simulink model "ex2_model"  (R2013a)
settings: Solver=ode45  StartTime=0.0  StopTime=10.0  RelTol=1e-3
values from neighbouring files (symbols this model uses):
  q_0 = 0    [ex6.m]
  q_dot_0 = 0    [ex6.m]
undefined symbols (not defined in the file or in its folder): q_dot_dot_0
settings Model: Creator=Brent  LastModifiedBy=Willdog

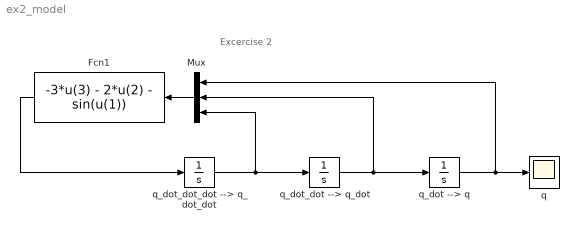
== system ex2_model ==
  note: Excercise 2
  Fcn1 : Fcn  Expr=-3*u(3) - 2*u(2) - sin(u(1))
  Mux : Mux  Inputs=3
  q : Scope
  q_dot --> q : Integrator  InitialCondition=q_0
  q_dot_dot --> q_dot : Integrator  InitialCondition=q_dot_0
  q_dot_dot_dot --> q_dot_dot : Integrator  InitialCondition=q_dot_dot_0
  wires:
  q_dot_dot --> q_dot/1 -> Mux/2, q_dot --> q/1
  q_dot_dot_dot --> q_dot_dot/1 -> Mux/3, q_dot_dot --> q_dot/1
  q_dot --> q/1 -> Mux/1, q/1
  Mux/1 -> Fcn1/1
  Fcn1/1 -> q_dot_dot_dot --> q_dot_dot/1
